simulink model "F16_Model_"  (R2025b)
settings: Solver=VariableStepAuto  StartTime=0.0  StopTime=100  RelTol=1e-3
values from neighbouring files (symbols this model uses):
  aero_data =     [aero_data.mat]
  b = 9.144    [initialization.m]
  c_bar = 3.45    [initialization.m]
  g = 9.81    [initialization.m]
  initial_pow = 50    [controlInputs.m]
  mass = 9295.4128    [initialization.m]
  S = 27.87    [initialization.m]
  u1 = 0    [controlInputs.m]
  u2 = 0    [controlInputs.m]
  u3 = -2    [controlInputs.m]
  u4 = 0    [controlInputs.m]
  u5 = 0    [controlInputs.m]
  u6 = 0.6    [controlInputs.m]
  xcg = 0.3*c_bar    (= 1.035)    [initialization.m]
  xcgr = 0.35*c_bar    (= 1.2075)    [initialization.m]
libraries: simulink_extras x9, aerolibfltsims x2, aerolibobsolete x1
(part 1 of 2)
settings Model: Creator=deepa  LastModifiedBy=deepa

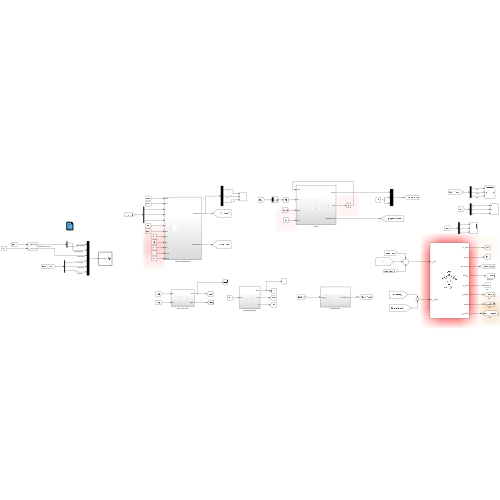
[thumbnail: Simulink's stored preview of the top-level diagram]
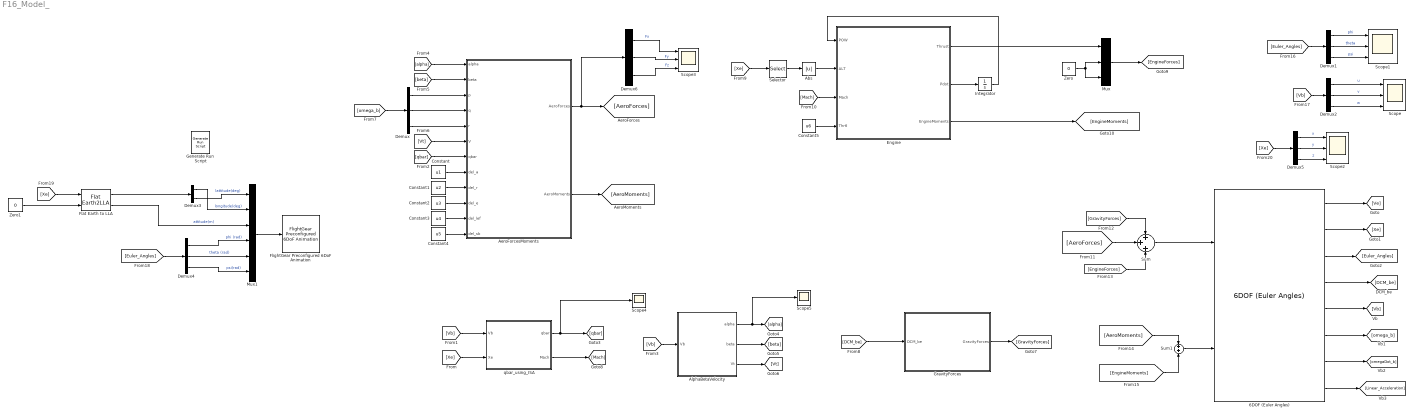
== system F16_Model_ ==
  6DOF (Euler Angles) : aerolibobsolete/6DOF (Euler Angles)  units=Metric (MKS)  mtype=Fixed  rep=Euler Angles  xme_0=[0 0 -1000]  Vm_0=[100 0 0]  eul_0=[0 0 0]  pm_0=[0 0 0]  mass_0=mass  mass_e=0.5  mass_f=2.0  inertia=I  inertia_e=eye(3)  inertia_f=2*eye(3)  k_quat=1.0  vre_flag=on  abi_flag=off  aMode=0  xme_statename=''  Vm_statename=''  eul_statename=''  quat_statename=''  pm_statename=''  mass_statename=''
  Abs : Abs  SaturateOnIntegerOverflow=off
  AeroForcesMoments : Subsystem
  AlphaBetaVelocity : Subsystem
  Constant : Constant  Value=u1
  Constant1 : Constant  Value=u2
  Constant2 : Constant  Value=u3
  Constant3 : Constant  Value=u4
  Constant4 : Constant  Value=u5
  Constant5 : Constant  Value=u6
  Demux{,1..2,4..6} (6 alike) : Demux  Outputs=3
  Demux3 : Demux  Outputs=2
  Engine : Subsystem
  Flat Earth to LLA : FlatEarth2LLA  R=6378137
  FlightGear Preconfigured 6DoF Animation : aerolibfltsims/FlightGear Preconfigured 6DoF Animation  xFlightGearVersion=v2019.1  DestinationIpAddress=127.0.0.1  DestinationPort=5502  SampleTime=1/30  packetVersion=24
  Generate Run Script : aerolibfltsims/Generate Run Script  Architecture=Win64  dataFlow=Send  GeometryModelName=c172p  AirportId=KSFO  RunwayId=10L  InitialAltitude=7224  InitialHeading=113  OffsetDistance=4.72  OffsetAzimuth=0  InstallScenery=off  DisableShaders=on  OriginAddress=127.0.0.1  DestinationPort=5502  OriginPort=5505  LocalAddress=127.0.0.1  OutputFileName=runfg.bat  FlightGearBaseDirectory=C:\Program Files\FlightGear 2024.1
  GravityForces : Subsystem
  Integrator : Integrator  InitialCondition=initial_pow
  Mux : Mux  Inputs=3
  Mux1 : Mux  Inputs=6
  Scope{,1..3} (4 alike) : Scope  NumInputPorts=3
      Scope settings: ActiveDisplayYMinimum=-502.98188581744421  ActiveDisplayYMaximum=2375.231294084077
      Scope1 settings: ActiveDisplayYMinimum=-1.0905728605767717  ActiveDisplayYMaximum=2.3543796241873545
      Scope2 settings: ActiveDisplayYMinimum=-88303.697025935631  ActiveDisplayYMaximum=46323.817378963853
      Scope3 settings: ActiveDisplayYMinimum=-6.05748400595E+6  ActiveDisplayYMaximum=3.40196349632E+6
  Scope4 : Scope
      settings: ActiveDisplayYMinimum=-166166.62177  ActiveDisplayYMaximum=1.49575944273E+6  DataLoggingVariableName=ScopeData2
  Scope5 : Scope
      settings: ActiveDisplayYMinimum=-7.38258  ActiveDisplayYMaximum=1.95471  DataLoggingVariableName=ScopeData3
  Selector : Selector  InputPortWidth=3  IndexOptions=Index vector (dialog)  Indices=3  OutputSizes=1
  Sum : Sum  Inputs=+++
  Sum1 : Sum
  Zero : Constant  Value=0  OutDataTypeStr=Inherit: Inherit via back propagation
  Zero1 : Constant  Value=0  OutDataTypeStr=Inherit: Inherit via back propagation
  qbar_using_ISA : Subsystem
  wires:
  6DOF (Euler Angles)/8 -> [Linear_Acceleration]
  6DOF (Euler Angles)/1 -> [Ve]
  6DOF (Euler Angles)/2 -> [Xe]
  6DOF (Euler Angles)/3 -> [Euler_Angles]
  6DOF (Euler Angles)/4 -> [DCM_be]
  6DOF (Euler Angles)/5 -> [Vb]
  6DOF (Euler Angles)/6 -> [omega_b]
  6DOF (Euler Angles)/7 -> [omegaDot_b]
  [Xe] -> qbar_using_ISA/2(Xe)
  [Vb] -> qbar_using_ISA/1(Vb)
  qbar_using_ISA/1(qbar) -> Scope4/1, [qbar]
  [qbar] -> AeroForcesMoments/7(qbar)
  [Vb] -> AlphaBetaVelocity/1(Vb)
  AlphaBetaVelocity/1(alpha) -> Scope5/1, [alpha]
  AlphaBetaVelocity/2(beta) -> [beta]
  AlphaBetaVelocity/3(Vt) -> [Vt]
  [alpha] -> AeroForcesMoments/1(alpha)
  [beta] -> AeroForcesMoments/2(beta)
  [Vt] -> AeroForcesMoments/6(V)
  [omega_b] -> Demux/1
  Demux/1 -> AeroForcesMoments/3(p)
  Demux/2 -> AeroForcesMoments/4(q)
  Demux/3 -> AeroForcesMoments/5(r)
  [DCM_be] -> GravityForces/1(DCM_be)
  GravityForces/1(GravityForces) -> [GravityForces]
  Engine/2(Pdot) -> Integrator/1
  Integrator/1 -> Engine/1(POW)
  [Xe] -> Selector/1
  Selector/1 -> Abs/1
  Abs/1 -> Engine/2(ALT)
  qbar_using_ISA/2(Mach) -> [Mach]
  [Mach] -> Engine/3(Mach)
  Engine/1(Thrust) -> Mux/1
  Mux/1 -> [EngineForces]
  Zero/1 -> Mux/2, Mux/3
  AeroForcesMoments/1(AeroForces) -> Demux6/1, [AeroForces]
  AeroForcesMoments/2(AeroMoments) -> [AeroMoments]
  [EngineForces] -> Sum/3
  [AeroForces] -> Sum/2
  [GravityForces] -> Sum/1
  Sum/1 -> 6DOF (Euler Angles)/1
  Engine/3(EngineMoments) -> [EngineMoments]
  [EngineMoments] -> Sum1/2
  [AeroMoments] -> Sum1/1
  Sum1/1 -> 6DOF (Euler Angles)/2
  Constant/1 -> AeroForcesMoments/8(del_a)
  Constant1/1 -> AeroForcesMoments/9(del_r)
  Constant2/1 -> AeroForcesMoments/10(del_e)
  Constant3/1 -> AeroForcesMoments/11(del_lef)
  Constant4/1 -> AeroForcesMoments/12(del_sb)
  Constant5/1 -> Engine/4(Thrtl)
  [Euler_Angles] -> Demux1/1
  Demux1/1 -> Scope1/1  "phi"
  Demux1/2 -> Scope1/2  "theta"
  Demux1/3 -> Scope1/3  "psi"
  [Vb] -> Demux2/1
  Demux2/1 -> Scope/1  "u"
  Demux2/2 -> Scope/2  "v"
  Demux2/3 -> Scope/3  "w"
  Flat Earth to LLA/1 -> Demux3/1
  Demux3/2 -> Mux1/1  "lattitude(deg)"
  Demux3/1 -> Mux1/2  "longitude(deg)"
  Flat Earth to LLA/2 -> Mux1/3  "attitude(m)"
  Demux4/1 -> Mux1/4  "phi (rad)"
  Demux4/2 -> Mux1/5  "theta (rad)"
  Demux4/3 -> Mux1/6  "psi(rad)"
  [Euler_Angles] -> Demux4/1
  Mux1/1 -> FlightGear Preconfigured 6DoF Animation/1
  [Xe] -> Flat Earth to LLA/1
  Zero1/1 -> Flat Earth to LLA/2
  [Xe] -> Demux5/1
  Demux5/1 -> Scope2/1  "x"
  Demux5/2 -> Scope2/2  "y"
  Demux5/3 -> Scope2/3  "z"
  Demux6/1 -> Scope3/1  "Fx"
  Demux6/2 -> Scope3/2  "Fy"
  Demux6/3 -> Scope3/3  "Fz"

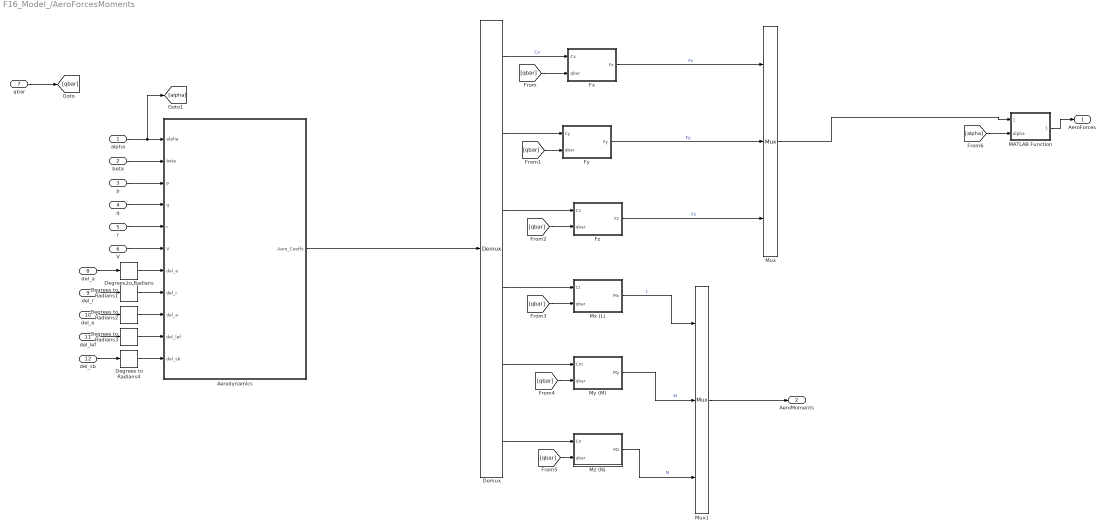
== system F16_Model_/AeroForcesMoments ==
  alpha : Inport
  beta : Inport  Port=2
  p : Inport  Port=3
  q : Inport  Port=4
  r : Inport  Port=5
  V : Inport  Port=6
  qbar : Inport  Port=7
  del_a : Inport  Port=8
  del_r : Inport  Port=9
  del_e : Inport  Port=10
  del_lef : Inport  Port=11
  del_sb : Inport  Port=12
  Aerodynamics : Subsystem
      mask Display: image('plane-8107709.jpg', [20,20,20,20,100,100]);
  Degrees to Radians{,1..4} (5 alike) : simulink_extras/Transformations/Degrees to Radians
  Demux : Demux  Outputs=6
  Fx : Subsystem
  Fy : Subsystem
  Fz : Subsystem
  MATLAB Function : MATLAB Function  TreatAsAtomicUnit=on
  Mux : Mux  Inputs=3
  Mux1 : Mux  Inputs=3
  Mx (L) : Subsystem
  My (M) : Subsystem
  Mz (N) : Subsystem
  AeroForces : Outport
  AeroMoments : Outport  Port=2
  wires:
  Aerodynamics/1(Aero_Coeffs) -> Demux/1
  Demux/3 -> Fz/1(Cz)
  Demux/5 -> My (M)/1(Cm)
  Demux/6 -> Mz (N)/1(Cn)
  Demux/2 -> Fy/1(Cy)
  Demux/4 -> Mx (L)/1(Cl)
  qbar/1 -> [qbar]
  Demux/1 -> Fx/1(Cx)  "Cx"
  Fx/1(Fx) -> Mux/1  "Fx"
  [qbar] -> Fx/2(qbar)
  [qbar] -> Fy/2(qbar)
  [qbar] -> Fz/2(qbar)
  [qbar] -> Mx (L)/2(qbar)
  [qbar] -> My (M)/2(qbar)
  [qbar] -> Mz (N)/2(qbar)
  Mx (L)/1(Mx) -> Mux1/1  "L"
  My (M)/1(My) -> Mux1/2  "M"
  Mz (N)/1(Mz) -> Mux1/3  "N"
  Mux/1 -> MATLAB Function/1(F_stability)
  Mux1/1 -> AeroMoments/1
  alpha/1 -> [alpha], Aerodynamics/1(alpha)
  beta/1 -> Aerodynamics/2(beta)
  p/1 -> Aerodynamics/3(p)
  q/1 -> Aerodynamics/4(q)
  r/1 -> Aerodynamics/5(r)
  V/1 -> Aerodynamics/6(V)
  del_a/1 -> Degrees to Radians/1
  del_r/1 -> Degrees to Radians1/1
  del_e/1 -> Degrees to Radians2/1
  del_lef/1 -> Degrees to Radians3/1
  del_sb/1 -> Degrees to Radians4/1
  Degrees to Radians/1 -> Aerodynamics/7(del_a)
  Degrees to Radians1/1 -> Aerodynamics/8(del_r)
  Degrees to Radians2/1 -> Aerodynamics/9(del_e)
  Degrees to Radians3/1 -> Aerodynamics/10(del_lef)
  Degrees to Radians4/1 -> Aerodynamics/11(del_sb)
  Fy/1(Fy) -> Mux/2  "Fy"
  Fz/1(Fz) -> Mux/3  "Fz"
  MATLAB Function/1(F_body) -> AeroForces/1
  [alpha] -> MATLAB Function/2(alpha)

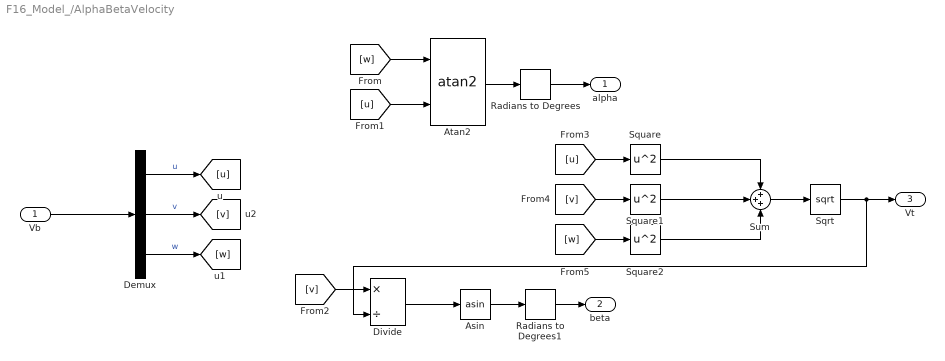
== system F16_Model_/AlphaBetaVelocity ==
  Vb : Inport
  Asin : Trigonometry  Operator=asin
  Atan2 : Trigonometry  Operator=atan2
  Demux : Demux  Outputs=3
  Divide : Product  Inputs=*/
  Radians to Degrees : simulink_extras/Transformations/Radians to Degrees
  Radians to Degrees1 : simulink_extras/Transformations/Radians to Degrees
  Sqrt : Sqrt
  Square : Math  Operator=square
  Square1 : Math  Operator=square
  Square2 : Math  Operator=square
  Sum : Sum  Inputs=+++
  alpha : Outport
  beta : Outport  Port=2
  Vt : Outport  Port=3
  wires:
  Vb/1 -> Demux/1
  Demux/1 -> [u]  "u"
  Demux/2 -> [v]  "v"
  Demux/3 -> [w]  "w"
  [u] -> Atan2/2
  [w] -> Atan2/1
  Atan2/1 -> Radians to Degrees/1
  [v] -> Divide/1
  Divide/1 -> Asin/1
  [u] -> Square/1
  [v] -> Square1/1
  [w] -> Square2/1
  Square/1 -> Sum/1
  Square1/1 -> Sum/2
  Square2/1 -> Sum/3
  Sum/1 -> Sqrt/1
  Sqrt/1 -> Divide/2, Vt/1
  Radians to Degrees/1 -> alpha/1
  Radians to Degrees1/1 -> beta/1
  Asin/1 -> Radians to Degrees1/1

== system F16_Model_/Engine ==
  POW : Inport
  ALT : Inport  Port=2
  Mach : Inport  Port=3
  Thrtl : Inport  Port=4
  Mux : Mux  Inputs=3
  PDOT : MATLAB Function  TreatAsAtomicUnit=on
  TGEAR : MATLAB Function  TreatAsAtomicUnit=on
  Thrust_ : MATLAB Function  TreatAsAtomicUnit=on
  Zero : Constant  Value=0  OutDataTypeStr=Inherit: Inherit via back propagation
  Thrust : Outport
  Pdot : Outport  Port=2
  EngineMoments : Outport  Port=3
  wires:
  Mach/1 -> Thrust_/3(MACH)
  POW/1 -> PDOT/1(P3), Thrust_/1(POW)
  Thrtl/1 -> TGEAR/1(THTL)
  TGEAR/1(TGEAR) -> PDOT/2(P1)
  PDOT/1(PDOT) -> Pdot/1
  ALT/1 -> Thrust_/2(ALT)
  Zero/1 -> Mux/3, Mux/2, Mux/1
  Mux/1 -> EngineMoments/1
  Thrust_/1(THRUST) -> Thrust/1

== system F16_Model_/GravityForces ==
  DCM_be : Inport
  Constant : Constant  Value=g
  Constant1 : Constant  Value=0
  Gain : Gain  Gain=mass
  Mux : Mux  Inputs=3
  Product : Product  Multiplication=Matrix(*)
  GravityForces : Outport
  wires:
  Constant/1 -> Gain/1
  Gain/1 -> Mux/3
  Constant1/1 -> Mux/2, Mux/1
  Mux/1 -> Product/2  "3x1"
  DCM_be/1 -> Product/1  "3x3"
  Product/1 -> GravityForces/1

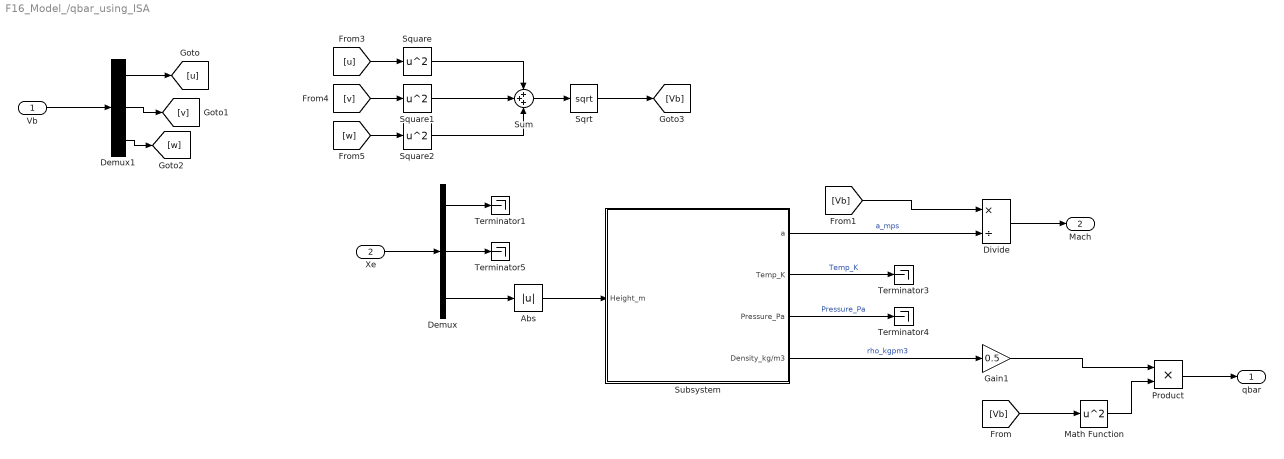
== system F16_Model_/qbar_using_ISA ==
  Vb : Inport
  Xe : Inport  Port=2
  Abs : Abs  SaturateOnIntegerOverflow=off
  Demux : Demux  Outputs=3
  Demux1 : Demux  Outputs=3
  Divide : Product  Inputs=*/
  Gain1 : Gain  Gain=0.5
  Math Function : Math  Operator=square
  Product : Product
  Sqrt : Sqrt
  Square : Math  Operator=square
  Square1 : Math  Operator=square
  Square2 : Math  Operator=square
  Subsystem : Subsystem
  Sum : Sum  Inputs=+++
  Terminator{1,3..5} (4 alike) : Terminator
  qbar : Outport
  Mach : Outport  Port=2
  wires:
  Subsystem/4(Density_kg/m3) -> Gain1/1  "rho_kgpm3"
  Subsystem/1(a) -> Divide/2  "a_mps"
  Subsystem/2(Temp_K) -> Terminator3/1  "Temp_K"
  Subsystem/3(Pressure_Pa) -> Terminator4/1  "Pressure_Pa"
  Gain1/1 -> Product/1
  Math Function/1 -> Product/2
  Product/1 -> qbar/1
  Xe/1 -> Demux/1
  Demux/1 -> Terminator1/1
  Demux/2 -> Terminator5/1
  Demux/3 -> Abs/1
  Vb/1 -> Demux1/1
  [Vb] -> Math Function/1
  [Vb] -> Divide/1
  Divide/1 -> Mach/1
  [v] -> Square1/1
  [w] -> Square2/1
  [u] -> Square/1
  Sum/1 -> Sqrt/1
  Square2/1 -> Sum/3
  Square/1 -> Sum/1
  Square1/1 -> Sum/2
  Sqrt/1 -> [Vb]
  Demux1/1 -> [u]
  Demux1/2 -> [v]
  Demux1/3 -> [w]
  Abs/1 -> Subsystem/1(Height_m)

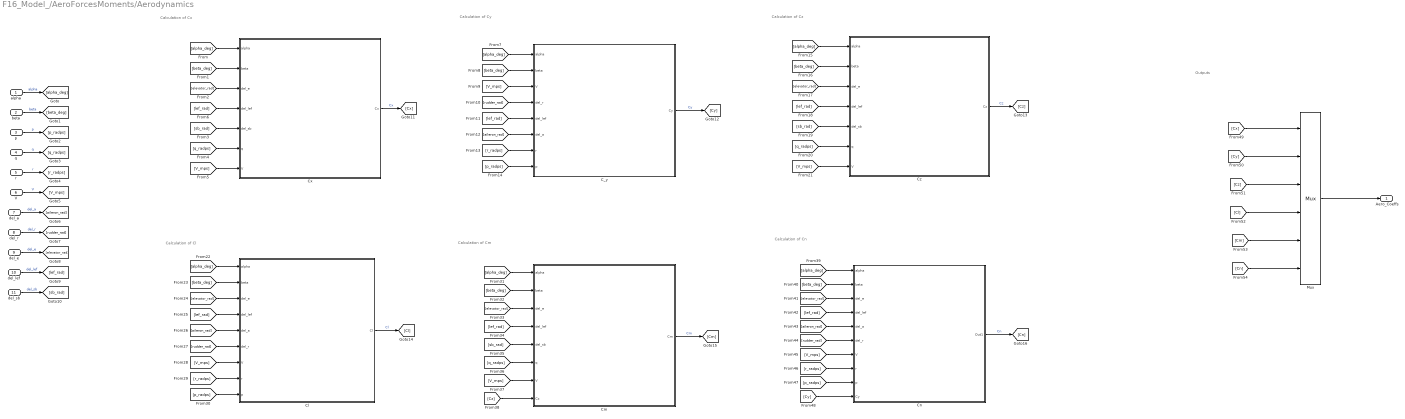
== system F16_Model_/AeroForcesMoments/Aerodynamics ==
  note: Outputs
  note: Calculation of Cn
  note: Calculation of Cm
  note: Calculation of Cl
  note: Calculation of Cy
  note: Calculation of Cx
  note: Calculation of Cz
  alpha : Inport
  beta : Inport  Port=2
  p : Inport  Port=3
  q : Inport  Port=4
  r : Inport  Port=5
  V : Inport  Port=6
  del_a : Inport  Port=7
  del_r : Inport  Port=8
  del_e : Inport  Port=9
  del_lef : Inport  Port=10
  del_sb : Inport  Port=11
  C_y : Subsystem
  Cl : Subsystem
  Cm : Subsystem
  Cn : Subsystem
  Cx : Subsystem
  Cz : Subsystem
  Mux : Mux  Inputs=6
  Aero_Coeffs : Outport
  wires:
  Mux/1 -> Aero_Coeffs/1
  alpha/1 -> [alpha_deg]  "alpha"
  beta/1 -> [beta_deg]  "beta"
  p/1 -> [p_radps]  "p"
  q/1 -> [q_radps]  "q"
  r/1 -> [r_radps]  "r"
  V/1 -> [V_mps]  "V"
  del_a/1 -> [aileron_rad]  "del_a"
  del_r/1 -> [rudder_rad]  "del_r"
  del_e/1 -> [elevator_rad]  "del_e"
  del_lef/1 -> [lef_rad]  "del_lef"
  del_sb/1 -> [sb_rad]  "del_sb"
  [alpha_deg] -> Cx/1(alpha)
  [beta_deg] -> Cx/2(beta)
  [elevator_rad] -> Cx/3(del_e)
  [lef_rad] -> Cx/4(del_lef)
  [sb_rad] -> Cx/5(del_sb)
  [q_radps] -> Cx/6(q)
  [V_mps] -> Cx/7(V)
  Cx/1(Cx) -> [Cx]  "Cx"
  [alpha_deg] -> C_y/1(alpha)
  [beta_deg] -> C_y/2(beta)
  [V_mps] -> C_y/3(V)
  [rudder_rad] -> C_y/4(del_r)
  [lef_rad] -> C_y/5(del_lef)
  [aileron_rad] -> C_y/6(del_a)
  [r_radps] -> C_y/7(r)
  [p_radps] -> C_y/8(p)
  C_y/1(Cy) -> [Cy]  "Cy"
  [alpha_deg] -> Cz/1(alpha)
  [beta_deg] -> Cz/2(beta)
  [elevator_rad] -> Cz/3(del_e)
  [lef_rad] -> Cz/4(del_lef)
  [sb_rad] -> Cz/5(del_sb)
  [q_radps] -> Cz/6(q)
  [V_mps] -> Cz/7(V)
  Cz/1(Cz) -> [Cz]  "Cz"
  [alpha_deg] -> Cl/1(alpha)
  [beta_deg] -> Cl/2(beta)
  [elevator_rad] -> Cl/3(del_e)
  [lef_rad] -> Cl/4(del_lef)
  [aileron_rad] -> Cl/5(del_a)
  [rudder_rad] -> Cl/6(del_r)
  [V_mps] -> Cl/7(V)
  [r_radps] -> Cl/8(r)
  [p_radps] -> Cl/9(p)
  Cl/1(Cl) -> [Cl]  "Cl"
  [alpha_deg] -> Cm/1(alpha)
  [beta_deg] -> Cm/2(beta)
  [elevator_rad] -> Cm/3(del_e)
  [lef_rad] -> Cm/4(del_lef)
  [sb_rad] -> Cm/5(del_sb)
  [q_radps] -> Cm/6(q)
  [V_mps] -> Cm/7(V)
  [Cz] -> Cm/8(Cz)
  Cm/1(Cm) -> [Cm]  "Cm"
  [alpha_deg] -> Cn/1(alpha)
  [beta_deg] -> Cn/2(beta)
  [elevator_rad] -> Cn/3(del_e)
  [lef_rad] -> Cn/4(del_lef)
  [aileron_rad] -> Cn/5(del_a)
  [rudder_rad] -> Cn/6(del_r)
  [V_mps] -> Cn/7(V)
  [r_radps] -> Cn/8(r)
  [p_radps] -> Cn/9(p)
  [Cy] -> Cn/10(Cy)
  Cn/1(Out1) -> [Cn]  "Cn"
  [Cx] -> Mux/1
  [Cy] -> Mux/2
  [Cz] -> Mux/3
  [Cl] -> Mux/4
  [Cm] -> Mux/5
  [Cn] -> Mux/6

== system F16_Model_/AeroForcesMoments/Fx ==
  Cx : Inport
  qbar : Inport  Port=2
  Gain : Gain  Gain=S
  Product : Product
  Fx : Outport
  wires:
  Product/1 -> Fx/1
  Gain/1 -> Product/1
  qbar/1 -> Product/2
  Cx/1 -> Gain/1

== system F16_Model_/AeroForcesMoments/Fy ==
  Cy : Inport
  qbar : Inport  Port=2
  Gain : Gain  Gain=S
  Product : Product
  Fy : Outport
  wires:
  Cy/1 -> Gain/1
  qbar/1 -> Product/2
  Gain/1 -> Product/1
  Product/1 -> Fy/1

== system F16_Model_/AeroForcesMoments/Fz ==
  Cz : Inport
  qbar : Inport  Port=2
  Gain : Gain  Gain=S
  Product : Product
  Fz : Outport
  wires:
  Product/1 -> Fz/1
  Gain/1 -> Product/1
  qbar/1 -> Product/2
  Cz/1 -> Gain/1

== system F16_Model_/AeroForcesMoments/Mx (L) ==
  Cl : Inport
  qbar : Inport  Port=2
  Gain : Gain  Gain=S*b
  Product : Product
  Mx : Outport
  wires:
  Cl/1 -> Gain/1
  qbar/1 -> Product/2
  Gain/1 -> Product/1
  Product/1 -> Mx/1

== system F16_Model_/AeroForcesMoments/My (M) ==
  Cm : Inport
  qbar : Inport  Port=2
  Gain : Gain  Gain=S*c_bar
  Product : Product
  My : Outport
  wires:
  Product/1 -> My/1
  Gain/1 -> Product/1
  qbar/1 -> Product/2
  Cm/1 -> Gain/1

== system F16_Model_/AeroForcesMoments/Mz (N) ==
  Cn : Inport
  qbar : Inport  Port=2
  Gain : Gain  Gain=S*b
  Product : Product
  Mz : Outport
  wires:
  Cn/1 -> Gain/1
  qbar/1 -> Product/2
  Gain/1 -> Product/1
  Product/1 -> Mz/1

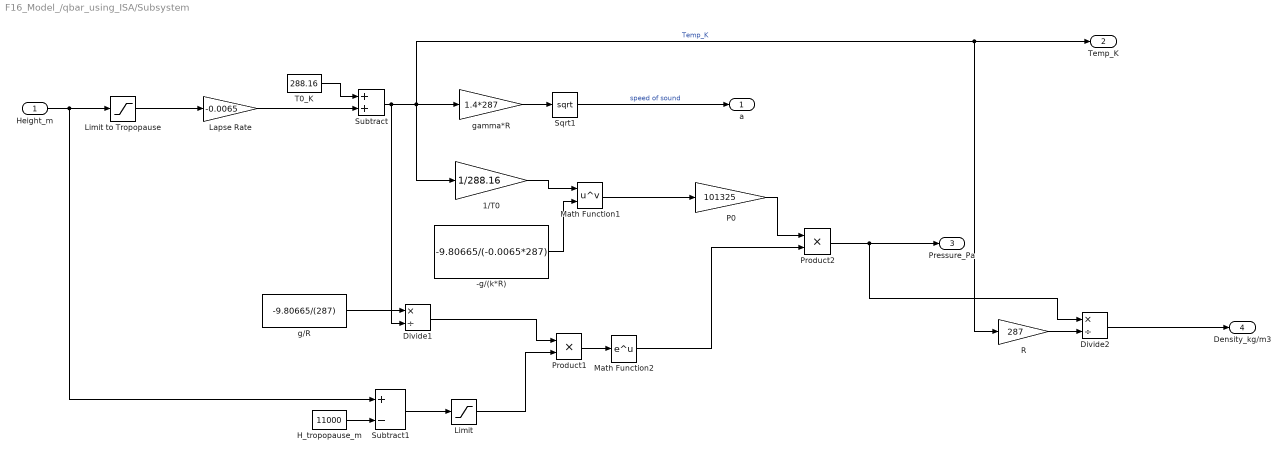
== system F16_Model_/qbar_using_ISA/Subsystem ==
  Height_m : Inport
  -g/(k*R) : Constant  Value=-9.80665/(-0.0065*287)
  1/T0 : Gain  Gain=1/288.16
  Divide1 : Product  Inputs=*/
  Divide2 : Product  Inputs=*/
  H_tropopause_m : Constant  Value=11000
  Lapse Rate : Gain  Gain=-0.0065
  "Limit " : Saturate  UpperLimit=inf  LowerLimit=0
  Limit to Tropopause : Saturate  UpperLimit=11000  LowerLimit=0
  Math Function1 : Math  Operator=pow
  Math Function2 : Math
  P0 : Gain  Gain=101325
  Product1 : Product
  Product2 : Product
  "R " : Gain  Gain=287
  Sqrt1 : Sqrt
  Subtract : Sum
  Subtract1 : Sum  Inputs=+-
  T0_K : Constant  Value=288.16
  g/R : Constant  Value=-9.80665/(287)
  gamma*R : Gain  Gain=1.4*287
  a : Outport
  Temp_K : Outport  Port=2
  Pressure_Pa : Outport  Port=3
  Density_kg/m3 : Outport  Port=4
  wires:
  1/T0/1 -> Math Function1/1
  H_tropopause_m/1 -> Subtract1/2
  P0/1 -> Product2/1
  Subtract/1 -> Divide1/2, gamma*R/1, 1/T0/1, Temp_K/1, "R "/1  "Temp_K"
  Lapse Rate/1 -> Subtract/2
  "R "/1 -> Divide2/2
  gamma*R/1 -> Sqrt1/1
  Limit to Tropopause/1 -> Lapse Rate/1
  T0_K/1 -> Subtract/1
  g/R/1 -> Divide1/1
  Product1/1 -> Math Function2/1
  Divide1/1 -> Product1/1
  Sqrt1/1 -> a/1  "speed of sound"
  Math Function1/1 -> P0/1
  Divide2/1 -> Density_kg/m3/1
  Product2/1 -> Pressure_Pa/1, Divide2/1
  Subtract1/1 -> "Limit "/1
  Height_m/1 -> Subtract1/1, Limit to Tropopause/1
  -g/(k*R)/1 -> Math Function1/2
  "Limit "/1 -> Product1/2
  Math Function2/1 -> Product2/2

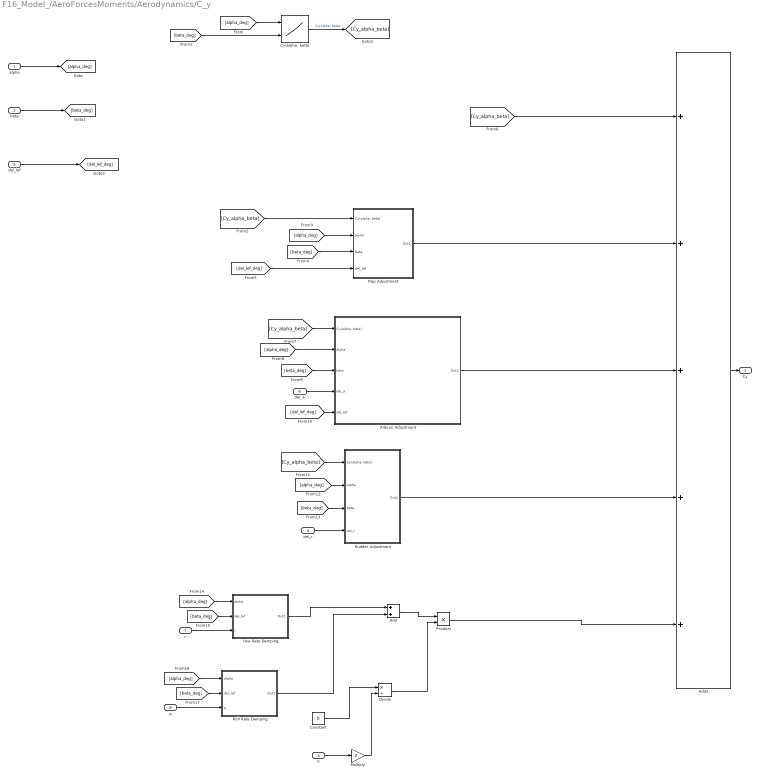
== system F16_Model_/AeroForcesMoments/Aerodynamics/C_y ==
  alpha : Inport
  beta : Inport  Port=2
  V : Inport  Port=3
  del_r : Inport  Port=4
  del_lef : Inport  Port=5
  del_a : Inport  Port=6
  r : Inport  Port=7
  p : Inport  Port=8
  Add : Sum
  Add2 : Sum  Inputs=+++++
  Aileron Adjustment : Subsystem
  Constant : Constant  Value=b
  "Cy(alpha, beta)" : Lookup_n-D  BreakpointsForDimension1=[-20, -15, -10, -5, 0, 5, 10, 15, 20, 25, 30, 35, 40, 45, 50, 55, 60, 70, 80, 90];  BreakpointsForDimension2=[-30, -25, -20, -15, -10, -8, -6, -4, -2, 0, 2, 4, 6, 8, 10, 15, 20, 25, 30];  Table=aero_data.Cy_alpha_beta  InternalRulePriority=Speed  RndMeth=Simplest
      settings: InputPortMap=u0,u1
  Divide : Product  Inputs=*/
  Flap Adjustment : Subsystem
  Multiply : Gain  Gain=2
  Product : Product
  Roll Rate Damping : Subsystem
  Rudder Adjustment : Subsystem
  Yaw Rate Damping : Subsystem
  Cy : Outport
  wires:
  Product/1 -> Add2/5
  Roll Rate Damping/1(Out1) -> Add/2
  Add/1 -> Product/1
  del_r/1 -> Rudder Adjustment/4(del_r)
  Yaw Rate Damping/1(Out1) -> Add/1
  p/1 -> Roll Rate Damping/3(p)
  Add2/1 -> Cy/1
  r/1 -> Yaw Rate Damping/3(r)
  del_a/1 -> Aileron Adjustment/4(del_a)
  Divide/1 -> Product/2
  Aileron Adjustment/1(Out1) -> Add2/3
  V/1 -> Multiply/1
  Flap Adjustment/1(Out1) -> Add2/2
  Rudder Adjustment/1(Out1) -> Add2/4
  Constant/1 -> Divide/1
  Multiply/1 -> Divide/2
  alpha/1 -> [alpha_deg]
  beta/1 -> [beta_deg]
  [alpha_deg] -> "Cy(alpha, beta)"/1
  [beta_deg] -> "Cy(alpha, beta)"/2
  "Cy(alpha, beta)"/1 -> [Cy_alpha_beta]  "Cy(alpha, beta)"
  [Cy_alpha_beta] -> Flap Adjustment/1("Cy(alpha, beta)")
  [alpha_deg] -> Flap Adjustment/2(alpha)
  [beta_deg] -> Flap Adjustment/3(beta)
  del_lef/1 -> [del_lef_deg]
  [del_lef_deg] -> Flap Adjustment/4(del_lef)
  [Cy_alpha_beta] -> Add2/1
  [Cy_alpha_beta] -> Aileron Adjustment/1("Cy(alpha, beta)")
  [alpha_deg] -> Aileron Adjustment/2(alpha)
  [beta_deg] -> Aileron Adjustment/3(beta)
  [del_lef_deg] -> Aileron Adjustment/5(del_lef)
  [Cy_alpha_beta] -> Rudder Adjustment/1("Cy(alpha, beta)")
  [alpha_deg] -> Rudder Adjustment/2(alpha)
  [beta_deg] -> Rudder Adjustment/3(beta)
  [alpha_deg] -> Yaw Rate Damping/1(alpha)
  [beta_deg] -> Yaw Rate Damping/2(del_lef)
  [alpha_deg] -> Roll Rate Damping/1(alpha)
  [beta_deg] -> Roll Rate Damping/2(del_lef)

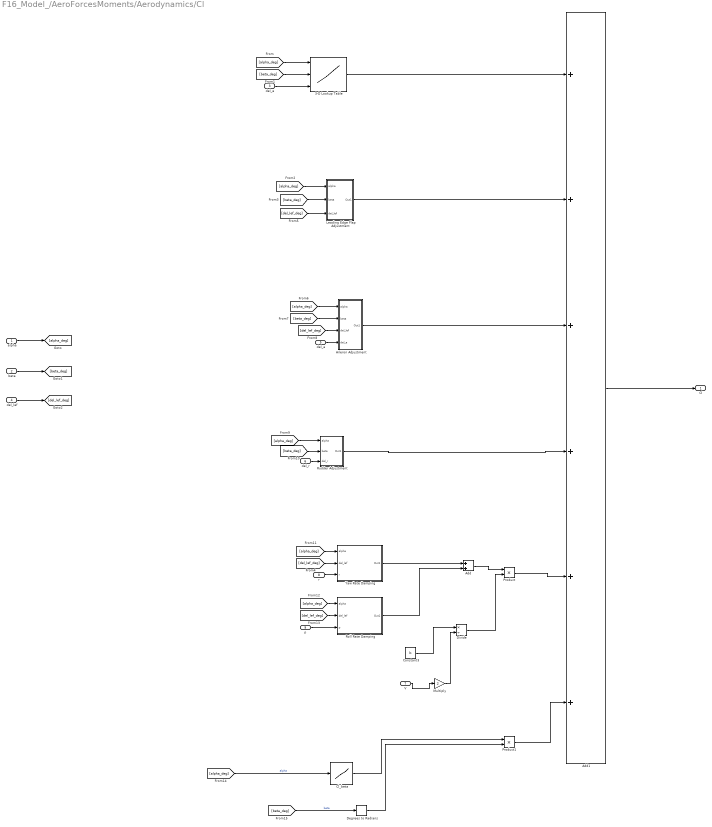
== system F16_Model_/AeroForcesMoments/Aerodynamics/Cl ==
  alpha : Inport
  beta : Inport  Port=2
  del_e : Inport  Port=3
  del_lef : Inport  Port=4
  del_a : Inport  Port=5
  del_r : Inport  Port=6
  V : Inport  Port=7
  r : Inport  Port=8
  p : Inport  Port=9
  3-D Lookup Table : Lookup_n-D  NumberOfTableDimensions=3  BreakpointsForDimension1=[-20, -15, -10, -5, 0, 5, 10, 15, 20, 25, 30, 35, 40, 45, 50, 55, 60, 70, 80, 90];  BreakpointsForDimension2=[-30, -25, -20, -15, -10, -8, -6, -4, -2, 0, 2, 4, 6, 8, 10, 15, 20, 25, 30];  BreakpointsForDimension3=[-25,0,25];  Table=aero_data.Cl_del_h  InternalRulePriority=Speed  RndMeth=Simplest
      settings: InputPortMap=u0,u1,u2
  Add : Sum
  Add1 : Sum  Inputs=++++++
  Aileron Adjustment : Subsystem
  Cl_beta : Lookup_n-D  NumberOfTableDimensions=1  BreakpointsForDimension1=[-20, -15, -10, -5, 0, 5, 10, 15, 20, 25, 30, 35, 40, 45, 50, 55, 60, 70, 80, 90];  Table=aero_data.del_Cl_beta  InternalRulePriority=Speed  RndMeth=Simplest
  Constant3 : Constant  Value=b
  Degrees to Radians : simulink_extras/Transformations/Degrees to Radians
  Divide : Product  Inputs=*/
  Leading Edge Flap Adjustment : Subsystem
  Multiply : Gain  Gain=2
  Product : Product
  Product1 : Product
  Roll Rate Damping : Subsystem
  Rudder Adjustment : Subsystem
  Yaw Rate Damping : Subsystem
  Cl : Outport
  wires:
  r/1 -> Yaw Rate Damping/3(r)
  Roll Rate Damping/1(Out1) -> Add/2
  del_r/1 -> Rudder Adjustment/3(del_r)
  Multiply/1 -> Divide/2
  Product/1 -> Add1/5
  p/1 -> Roll Rate Damping/3(p)
  del_a/1 -> Aileron Adjustment/4(del_a)
  3-D Lookup Table/1 -> Add1/1
  Constant3/1 -> Divide/1
  Rudder Adjustment/1(Out1) -> Add1/4
  Add1/1 -> Cl/1
  Leading Edge Flap Adjustment/1(Out1) -> Add1/2
  Yaw Rate Damping/1(Out1) -> Add/1
  Add/1 -> Product/1
  V/1 -> Multiply/1
  Divide/1 -> Product/2
  Cl_beta/1 -> Product1/1
  Degrees to Radians/1 -> Product1/2
  Product1/1 -> Add1/6
  [beta_deg] -> Degrees to Radians/1  "beta"
  [alpha_deg] -> Cl_beta/1  "alpha"
  alpha/1 -> [alpha_deg]
  beta/1 -> [beta_deg]
  [alpha_deg] -> 3-D Lookup Table/1
  [beta_deg] -> 3-D Lookup Table/2
  del_e/1 -> 3-D Lookup Table/3
  [alpha_deg] -> Leading Edge Flap Adjustment/1(alpha)
  [beta_deg] -> Leading Edge Flap Adjustment/2(beta)
  del_lef/1 -> [del_lef_deg]
  [del_lef_deg] -> Yaw Rate Damping/2(del_lef)
  [del_lef_deg] -> Leading Edge Flap Adjustment/3(del_lef)
  [alpha_deg] -> Aileron Adjustment/1(alpha)
  [beta_deg] -> Aileron Adjustment/2(beta)
  [del_lef_deg] -> Aileron Adjustment/3(del_lef)
  [alpha_deg] -> Rudder Adjustment/1(alpha)
  [beta_deg] -> Rudder Adjustment/2(beta)
  [alpha_deg] -> Yaw Rate Damping/1(alpha)
  [alpha_deg] -> Roll Rate Damping/1(alpha)
  [del_lef_deg] -> Roll Rate Damping/2(del_lef)
  Aileron Adjustment/1(Out1) -> Add1/3

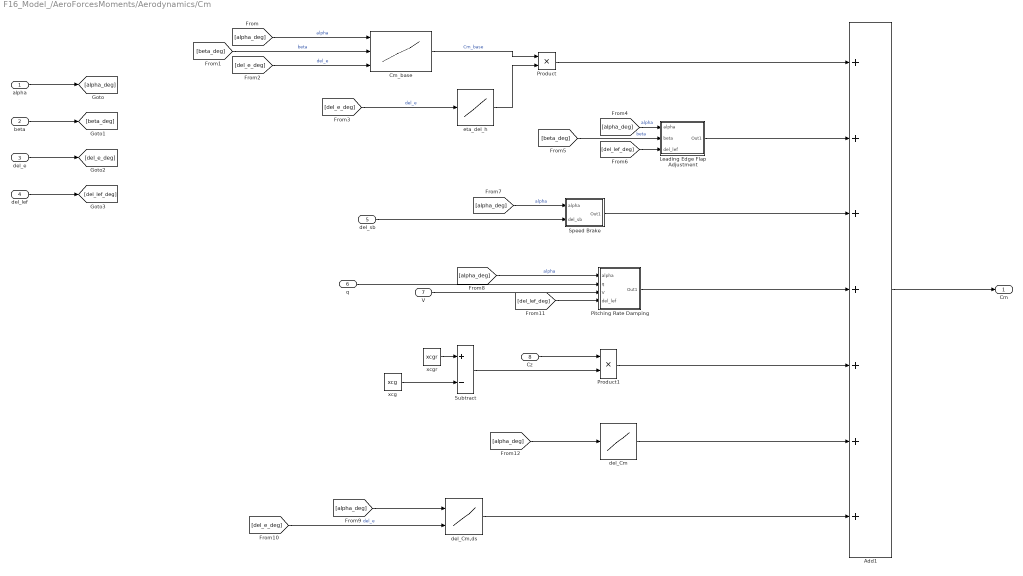
== system F16_Model_/AeroForcesMoments/Aerodynamics/Cm ==
  alpha : Inport
  beta : Inport  Port=2
  del_e : Inport  Port=3
  del_lef : Inport  Port=4
  del_sb : Inport  Port=5
  q : Inport  Port=6
  V : Inport  Port=7
  Cz : Inport  Port=8
  " Cm_base" : Lookup_n-D  NumberOfTableDimensions=3  BreakpointsForDimension1=[-20, -15, -10, -5, 0, 5, 10, 15, 20, 25, 30, 35, 40, 45, 50, 55, 60, 70, 80, 90];  BreakpointsForDimension2=[-30, -25, -20, -15, -10, -8, -6, -4, -2, 0, 2, 4, 6, 8, 10, 15, 20, 25, 30];  BreakpointsForDimension3=[-25, -10, 0, 10, 25]  Table=aero_data.Cm_del_h  InternalRulePriority=Speed  RndMeth=Simplest
      settings: InputPortMap=u0,u1,u2
  Add1 : Sum  Inputs=+++++++
  Leading Edge Flap Adjustment : Subsystem
  Pitching Rate Damping : Subsystem
  Product : Product
  Product1 : Product
  Speed Brake : Subsystem
  Subtract : Sum  Inputs=+-
  del_Cm : Lookup_n-D  NumberOfTableDimensions=1  BreakpointsForDimension1=[-20, -15, -10, -5, 0, 5, 10, 15, 20, 25, 30, 35, 40, 45, 50, 55, 60, 70, 80, 90]  Table=aero_data.del_Cm  InternalRulePriority=Speed  RndMeth=Simplest
  del_Cm,ds : Lookup_n-D  BreakpointsForDimension1=[-20, -15, -10, -5, 0, 5, 10, 15, 20, 25, 30, 35, 40, 45, 50, 55, 60, 70, 80, 90];  BreakpointsForDimension2=[-25, -10, 0, 10, 15, 20, 25]  Table=aero_data.del_Cm_ds  InternalRulePriority=Speed  RndMeth=Simplest
      settings: InputPortMap=u0,u1
  eta_del_h : Lookup_n-D  NumberOfTableDimensions=1  BreakpointsForDimension1=[-25, -10, 0, 10, 25]  Table=aero_data.eta_del_h  InternalRulePriority=Speed  RndMeth=Simplest
  xcg : Constant  Value=xcg
  xcgr : Constant  Value=xcgr
  Cm : Outport
  wires:
  Speed Brake/1(Out1) -> Add1/3
  Pitching Rate Damping/1(Out1) -> Add1/4
  Leading Edge Flap Adjustment/1(Out1) -> Add1/2
  Add1/1 -> Cm/1
  del_sb/1 -> Speed Brake/2(del_sb)
  q/1 -> Pitching Rate Damping/2(q)
  V/1 -> Pitching Rate Damping/3(V)
  " Cm_base"/1 -> Product/1  "Cm_base"
  eta_del_h/1 -> Product/2
  Product/1 -> Add1/1
  Cz/1 -> Product1/1
  xcgr/1 -> Subtract/1
  xcg/1 -> Subtract/2
  Subtract/1 -> Product1/2
  Product1/1 -> Add1/5
  del_Cm/1 -> Add1/6
  del_Cm,ds/1 -> Add1/7
  [alpha_deg] -> " Cm_base"/1  "alpha"
  [beta_deg] -> " Cm_base"/2  "beta"
  [del_e_deg] -> eta_del_h/1  "del_e"
  [del_e_deg] -> " Cm_base"/3  "del_e"
  alpha/1 -> [alpha_deg]
  beta/1 -> [beta_deg]
  del_e/1 -> [del_e_deg]
  del_lef/1 -> [del_lef_deg]
  [alpha_deg] -> Leading Edge Flap Adjustment/1(alpha)  "alpha"
  [beta_deg] -> Leading Edge Flap Adjustment/2(beta)  "beta"
  [del_lef_deg] -> Leading Edge Flap Adjustment/3(del_lef)
  [alpha_deg] -> Speed Brake/1(alpha)  "alpha"
  [alpha_deg] -> Pitching Rate Damping/1(alpha)  "alpha"
  [alpha_deg] -> del_Cm,ds/1
  [del_e_deg] -> del_Cm,ds/2  "del_e"
  [del_lef_deg] -> Pitching Rate Damping/4(del_lef)
  [alpha_deg] -> del_Cm/1

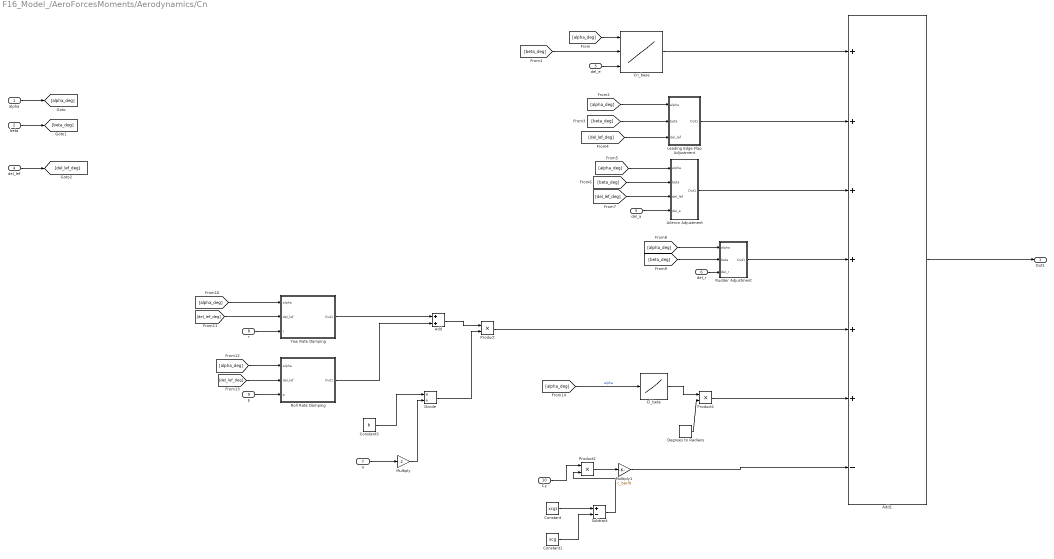
== system F16_Model_/AeroForcesMoments/Aerodynamics/Cn ==
  alpha : Inport
  beta : Inport  Port=2
  del_e : Inport  Port=3
  del_lef : Inport  Port=4
  del_a : Inport  Port=5
  del_r : Inport  Port=6
  V : Inport  Port=7
  r : Inport  Port=8
  p : Inport  Port=9
  Cy : Inport  Port=10
  Add : Sum
  Add1 : Sum  Inputs=++++++-
  Aileron Adjustment : Subsystem
  Cl_beta : Lookup_n-D  NumberOfTableDimensions=1  BreakpointsForDimension1=[-20, -15, -10, -5, 0, 5, 10, 15, 20, 25, 30, 35, 40, 45, 50, 55, 60, 70, 80, 90];  Table=aero_data.del_Cn_beta  InternalRulePriority=Speed  RndMeth=Simplest
  Cn_base : Lookup_n-D  NumberOfTableDimensions=3  BreakpointsForDimension1=[-20, -15, -10, -5, 0, 5, 10, 15, 20, 25, 30, 35, 40, 45, 50, 55, 60, 70, 80, 90];  BreakpointsForDimension2=[-30, -25, -20, -15, -10, -8, -6, -4, -2, 0, 2, 4, 6, 8, 10, 15, 20, 25, 30];  BreakpointsForDimension3=[-25,0,25];  Table=aero_data.Cn_del_h  InternalRulePriority=Speed  RndMeth=Simplest
      settings: InputPortMap=u0,u1,u2
  Constant : Constant  Value=xcgr
  Constant1 : Constant  Value=xcg
  Constant3 : Constant  Value=b
  Degrees to Radians : simulink_extras/Transformations/Degrees to Radians
  Divide : Product  Inputs=*/
  Leading Edge Flap Adjustment : Subsystem
  Multiply : Gain  Gain=2
  Multiply1 : Gain  Gain=c_bar/b
  Product : Product
  Product1 : Product
  Product2 : Product
  Roll Rate Damping : Subsystem
  Rudder Adjustment : Subsystem
  Subtract : Sum  Inputs=+-
  Yaw Rate Damping : Subsystem
  Out1 : Outport
  wires:
  r/1 -> Yaw Rate Damping/3(r)
  Roll Rate Damping/1(Out1) -> Add/2
  del_r/1 -> Rudder Adjustment/3(del_r)
  Aileron Adjustment/1(Out1) -> Add1/3
  Multiply/1 -> Divide/2
  Product/1 -> Add1/5
  p/1 -> Roll Rate Damping/3(p)
  del_a/1 -> Aileron Adjustment/4(del_a)
  Cn_base/1 -> Add1/1
  Constant3/1 -> Divide/1
  Rudder Adjustment/1(Out1) -> Add1/4
  Add1/1 -> Out1/1
  Leading Edge Flap Adjustment/1(Out1) -> Add1/2
  Yaw Rate Damping/1(Out1) -> Add/1
  del_e/1 -> Cn_base/3
  Add/1 -> Product/1
  V/1 -> Multiply/1
  Divide/1 -> Product/2
  Cl_beta/1 -> Product1/1
  Degrees to Radians/1 -> Product1/2
  Product1/1 -> Add1/6
  Constant/1 -> Subtract/1
  Constant1/1 -> Subtract/2
  Cy/1 -> Product2/1
  Subtract/1 -> Product2/2
  Product2/1 -> Multiply1/1
  Multiply1/1 -> Add1/7
  [alpha_deg] -> Cl_beta/1  "alpha"
  alpha/1 -> [alpha_deg]
  beta/1 -> [beta_deg]
  del_lef/1 -> [del_lef_deg]
  [alpha_deg] -> Cn_base/1
  [beta_deg] -> Cn_base/2
  [alpha_deg] -> Leading Edge Flap Adjustment/1(alpha)
  [beta_deg] -> Leading Edge Flap Adjustment/2(beta)
  [del_lef_deg] -> Leading Edge Flap Adjustment/3(del_lef)
  [alpha_deg] -> Aileron Adjustment/1(alpha)
  [beta_deg] -> Aileron Adjustment/2(beta)
  [del_lef_deg] -> Aileron Adjustment/3(del_lef)
  [alpha_deg] -> Rudder Adjustment/1(alpha)
  [beta_deg] -> Rudder Adjustment/2(beta)
  [alpha_deg] -> Yaw Rate Damping/1(alpha)
  [del_lef_deg] -> Yaw Rate Damping/2(del_lef)
  [alpha_deg] -> Roll Rate Damping/1(alpha)
  [del_lef_deg] -> Roll Rate Damping/2(del_lef)

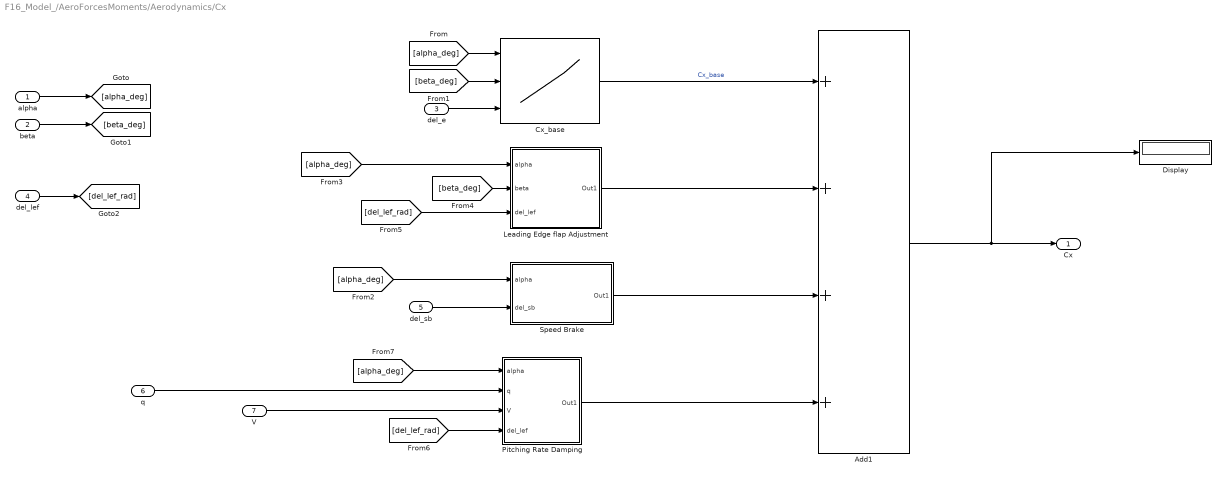
== system F16_Model_/AeroForcesMoments/Aerodynamics/Cx ==
  alpha : Inport
  beta : Inport  Port=2
  del_e : Inport  Port=3
  del_lef : Inport  Port=4
  del_sb : Inport  Port=5
  q : Inport  Port=6
  V : Inport  Port=7
  " Cx_base" : Lookup_n-D  NumberOfTableDimensions=3  BreakpointsForDimension1=[-20, -15, -10, -5, 0, 5, 10, 15, 20, 25, 30, 35, 40, 45, 50, 55, 60, 70, 80, 90];  BreakpointsForDimension2=[-30, -25, -20, -15, -10, -8, -6, -4, -2, 0, 2, 4, 6, 8, 10, 15, 20, 25, 30];  BreakpointsForDimension3=[-25, -10, 0, 10, 25];  Table=aero_data.Cx_del_h  InternalRulePriority=Speed  RndMeth=Simplest
      settings: InputPortMap=u0,u1,u2
  Add1 : Sum  Inputs=++++
  Display : Display
  Leading Edge flap Adjustment : Subsystem
  Pitching Rate Damping : Subsystem
  Speed Brake : Subsystem
  Cx : Outport
  wires:
  del_e/1 -> " Cx_base"/3
  Speed Brake/1(Out1) -> Add1/3
  " Cx_base"/1 -> Add1/1  "Cx_base"
  Pitching Rate Damping/1(Out1) -> Add1/4
  Leading Edge flap Adjustment/1(Out1) -> Add1/2
  Add1/1 -> Display/1, Cx/1
  del_sb/1 -> Speed Brake/2(del_sb)
  q/1 -> Pitching Rate Damping/2(q)
  V/1 -> Pitching Rate Damping/3(V)
  alpha/1 -> [alpha_deg]
  beta/1 -> [beta_deg]
  [alpha_deg] -> " Cx_base"/1
  [beta_deg] -> " Cx_base"/2
  del_lef/1 -> [del_lef_rad]
  [alpha_deg] -> Speed Brake/1(alpha)
  [alpha_deg] -> Leading Edge flap Adjustment/1(alpha)
  [beta_deg] -> Leading Edge flap Adjustment/2(beta)
  [del_lef_rad] -> Leading Edge flap Adjustment/3(del_lef)
  [del_lef_rad] -> Pitching Rate Damping/4(del_lef)
  [alpha_deg] -> Pitching Rate Damping/1(alpha)

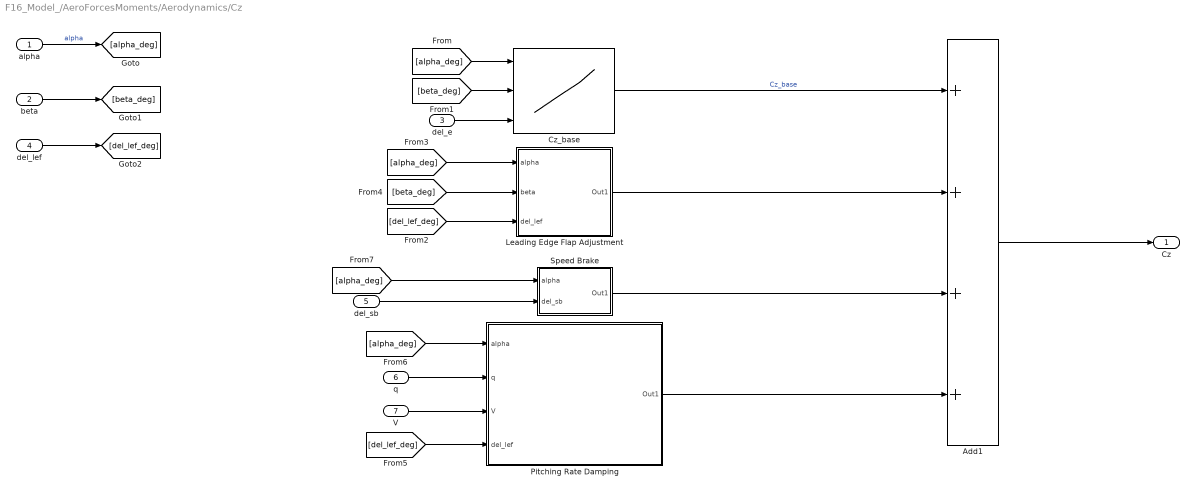
== system F16_Model_/AeroForcesMoments/Aerodynamics/Cz ==
  alpha : Inport
  beta : Inport  Port=2
  del_e : Inport  Port=3
  del_lef : Inport  Port=4
  del_sb : Inport  Port=5
  q : Inport  Port=6
  V : Inport  Port=7
  Add1 : Sum  Inputs=++++
  Cz_base : Lookup_n-D  NumberOfTableDimensions=3  BreakpointsForDimension1=[-20, -15, -10, -5, 0, 5, 10, 15, 20, 25, 30, 35, 40, 45, 50, 55, 60, 70, 80, 90];  BreakpointsForDimension2=[-30, -25, -20, -15, -10, -8, -6, -4, -2, 0, 2, 4, 6, 8, 10, 15, 20, 25, 30];  BreakpointsForDimension3=[-25, -10, 0, 10, 25];  Table=aero_data.Cz_del_h  InternalRulePriority=Speed  RndMeth=Simplest
      settings: InputPortMap=u0,u1,u2
  Leading Edge Flap Adjustment : Subsystem
  Pitching Rate Damping : Subsystem
  Speed Brake : Subsystem
  Cz : Outport
  wires:
  del_e/1 -> Cz_base/3
  Speed Brake/1(Out1) -> Add1/3
  Cz_base/1 -> Add1/1  "Cz_base"
  Pitching Rate Damping/1(Out1) -> Add1/4
  Leading Edge Flap Adjustment/1(Out1) -> Add1/2
  Add1/1 -> Cz/1
  del_sb/1 -> Speed Brake/2(del_sb)
  q/1 -> Pitching Rate Damping/2(q)
  V/1 -> Pitching Rate Damping/3(V)
  alpha/1 -> [alpha_deg]  "alpha"
  beta/1 -> [beta_deg]
  [alpha_deg] -> Cz_base/1
  [beta_deg] -> Cz_base/2
  del_lef/1 -> [del_lef_deg]
  [del_lef_deg] -> Leading Edge Flap Adjustment/3(del_lef)
  [alpha_deg] -> Leading Edge Flap Adjustment/1(alpha)
  [beta_deg] -> Leading Edge Flap Adjustment/2(beta)
  [del_lef_deg] -> Pitching Rate Damping/4(del_lef)
  [alpha_deg] -> Pitching Rate Damping/1(alpha)
  [alpha_deg] -> Speed Brake/1(alpha)

== system F16_Model_/AeroForcesMoments/Aerodynamics/C_y/Aileron Adjustment ==
  "Cy(alpha, beta)" : Inport
  alpha : Inport  Port=2
  beta : Inport  Port=3
  del_a : Inport  Port=4
  del_lef : Inport  Port=5
  Add1 : Sum
  Cy_del_a_20 : Lookup_n-D  BreakpointsForDimension1=[-20, -15, -10, -5, 0, 5, 10, 15, 20, 25, 30, 35, 40, 45, 50, 55, 60, 70, 80, 90];  BreakpointsForDimension2=[-30, -25, -20, -15, -10, -8, -6, -4, -2, 0, 2, 4, 6, 8, 10, 15, 20, 25, 30];  Table=aero_data.Cy_del_a_20  InternalRulePriority=Speed  RndMeth=Simplest
      settings: InputPortMap=u0,u1
  Multiply1 : Gain  Gain=0.05
  Product2 : Product
  Subtract1 : Sum  Inputs=-+
  del_Cy_del_a_20*(1-del_lef/25) : Subsystem
  Out1 : Outport
  wires:
  beta/1 -> Cy_del_a_20/2, del_Cy_del_a_20*(1-del_lef/25)/2(beta)
  Multiply1/1 -> Product2/2
  Add1/1 -> Product2/1
  Subtract1/1 -> Add1/1
  del_a/1 -> Multiply1/1
  Cy_del_a_20/1 -> Subtract1/2  "Cy_del_a_20"
  del_Cy_del_a_20*(1-del_lef/25)/1(Out1) -> Add1/2
  del_lef/1 -> del_Cy_del_a_20*(1-del_lef/25)/3(del_lef)
  Product2/1 -> Out1/1
  alpha/1 -> del_Cy_del_a_20*(1-del_lef/25)/1(alpha), Cy_del_a_20/1
  "Cy(alpha, beta)"/1 -> Subtract1/1

== system F16_Model_/AeroForcesMoments/Aerodynamics/C_y/Flap Adjustment ==
  "Cy(alpha, beta)" : Inport
  alpha : Inport  Port=2
  beta : Inport  Port=3
  del_lef : Inport  Port=4
  1-del_lef/25 : Subsystem
  Cy_lef : Lookup_n-D  BreakpointsForDimension1=[-20, -15, -10, -5, 0, 5, 10, 15, 20, 25, 30, 35, 40, 45];  BreakpointsForDimension2=[-30, -25, -20, -15, -10, -8, -6, -4, -2, 0, 2, 4, 6, 8, 10, 15, 20, 25, 30];  Table=aero_data.Cy_lef  InternalRulePriority=Speed  RndMeth=Simplest
      settings: InputPortMap=u0,u1
  Product3 : Product
  Subtract2 : Sum  Inputs=+-
  Out1 : Outport
  wires:
  "Cy(alpha, beta)"/1 -> Subtract2/2
  1-del_lef/25/1(1 - del_lef/25) -> Product3/2
  del_lef/1 -> 1-del_lef/25/1(del_lef1)
  Cy_lef/1 -> Subtract2/1  "Cy_lef"
  Subtract2/1 -> Product3/1
  alpha/1 -> Cy_lef/1
  beta/1 -> Cy_lef/2
  Product3/1 -> Out1/1

== system F16_Model_/AeroForcesMoments/Aerodynamics/C_y/Roll Rate Damping ==
  alpha : Inport
  del_lef : Inport  Port=2
  p : Inport  Port=3
  Add : Sum
  Constant : Constant
  Constant1 : Constant  Value=25
  Cy_p : Lookup_n-D  NumberOfTableDimensions=1  BreakpointsForDimension1=[-20, -15, -10, -5, 0, 5, 10, 15, 20, 25, 30, 35, 40, 45, 50, 55, 60, 70, 80, 90];  Table=aero_data.Cy_p  InternalRulePriority=Speed  RndMeth=Simplest
  Divide : Product  Inputs=*/
  Product : Product
  Product1 : Product
  Subtract : Sum  Inputs=+-
  del_Cy_p_lef : Lookup_n-D  NumberOfTableDimensions=1  BreakpointsForDimension1=[-20, -15, -10, -5, 0, 5, 10, 15, 20, 25, 30, 35, 40, 45];  Table=aero_data.del_Cy_p_lef  InternalRulePriority=Speed  RndMeth=Simplest
  Out1 : Outport
  wires:
  alpha/1 -> del_Cy_p_lef/1, Cy_p/1
  del_Cy_p_lef/1 -> Product/1  "del_Cy_p_lef"
  Cy_p/1 -> Add/1
  del_lef/1 -> Divide/1
  Constant1/1 -> Divide/2
  Constant/1 -> Subtract/1
  Divide/1 -> Subtract/2
  Subtract/1 -> Product/2  "1 - del_lef/25"
  Product/1 -> Add/2
  Add/1 -> Product1/1
  p/1 -> Product1/2
  Product1/1 -> Out1/1

== system F16_Model_/AeroForcesMoments/Aerodynamics/C_y/Rudder Adjustment ==
  "Cy(alpha, beta)" : Inport
  alpha : Inport  Port=2
  beta : Inport  Port=3
  del_r : Inport  Port=4
  Cy_del_r_30 : Lookup_n-D  BreakpointsForDimension1=[-20, -15, -10, -5, 0, 5, 10, 15, 20, 25, 30, 35, 40, 45, 50, 55, 60, 70, 80, 90];  BreakpointsForDimension2=[-30, -25, -20, -15, -10, -8, -6, -4, -2, 0, 2, 4, 6, 8, 10, 15, 20, 25, 30];  Table=aero_data.Cy_r_del_r_30  InternalRulePriority=Speed  RndMeth=Simplest
      settings: InputPortMap=u0,u1
  Product1 : Product
  Subtract : Sum  Inputs=+-
  Out1 : Outport
  wires:
  "Cy(alpha, beta)"/1 -> Subtract/2
  del_r/1 -> Product1/1
  Subtract/1 -> Product1/2
  Cy_del_r_30/1 -> Subtract/1  "Cy_del_r_30"
  alpha/1 -> Cy_del_r_30/1
  beta/1 -> Cy_del_r_30/2
  Product1/1 -> Out1/1

== system F16_Model_/AeroForcesMoments/Aerodynamics/C_y/Yaw Rate Damping ==
  alpha : Inport
  del_lef : Inport  Port=2
  r : Inport  Port=3
  Add : Sum
  Constant : Constant
  Constant1 : Constant  Value=25
  Cy_r : Lookup_n-D  NumberOfTableDimensions=1  BreakpointsForDimension1=[-20, -15, -10, -5, 0, 5, 10, 15, 20, 25, 30, 35, 40, 45, 50, 55, 60, 70, 80, 90];  Table=aero_data.Cy_r  InternalRulePriority=Speed  RndMeth=Simplest
  Divide : Product  Inputs=*/
  Product : Product
  Product1 : Product
  Subtract : Sum  Inputs=+-
  del_Cy_r_lef : Lookup_n-D  NumberOfTableDimensions=1  BreakpointsForDimension1=[-20, -15, -10, -5, 0, 5, 10, 15, 20, 25, 30, 35, 40, 45];  Table=aero_data.del_Cy_r_lef  InternalRulePriority=Speed  RndMeth=Simplest
  Out1 : Outport
  wires:
  Cy_r/1 -> Add/1
  alpha/1 -> del_Cy_r_lef/1, Cy_r/1
  del_Cy_r_lef/1 -> Product/1
  del_lef/1 -> Divide/1
  Divide/1 -> Subtract/2
  Subtract/1 -> Product/2  "1 - del_lef/25"
  Constant/1 -> Subtract/1
  Constant1/1 -> Divide/2
  Product/1 -> Add/2
  Add/1 -> Product1/1
  r/1 -> Product1/2
  Product1/1 -> Out1/1

== system F16_Model_/AeroForcesMoments/Aerodynamics/Cl/Aileron Adjustment ==
  alpha : Inport
  beta : Inport  Port=2
  del_lef : Inport  Port=3
  del_a : Inport  Port=4
  Add : Sum
  Cl_del_a_20 : Lookup_n-D  BreakpointsForDimension1=[-20, -15, -10, -5, 0, 5, 10, 15, 20, 25, 30, 35, 40, 45, 50, 55, 60, 70, 80, 90];  BreakpointsForDimension2=[-30, -25, -20, -15, -10, -8, -6, -4, -2, 0, 2, 4, 6, 8, 10, 15, 20, 25, 30];  Table=aero_data.Cl_del_a_20  InternalRulePriority=Speed  RndMeth=Simplest
      settings: InputPortMap=u0,u1
  Cl_del_a_20_lef : Lookup_n-D  BreakpointsForDimension1=[-20, -15, -10, -5, 0, 5, 10, 15, 20, 25, 30, 35, 40, 45];  BreakpointsForDimension2=[-30, -25, -20, -15, -10, -8, -6, -4, -2, 0, 2, 4, 6, 8, 10, 15, 20, 25, 30];  Table=aero_data.Cl_del_a_20_lef  InternalRulePriority=Speed  RndMeth=Simplest
      settings: InputPortMap=u0,u1
  Cl_del_h_0 : Lookup_n-D  BreakpointsForDimension1=[-20, -15, -10, -5, 0, 5, 10, 15, 20, 25, 30, 35, 40, 45, 50, 55, 60, 70, 80, 90];  BreakpointsForDimension2=[-30, -25, -20, -15, -10, -8, -6, -4, -2, 0, 2, 4, 6, 8, 10, 15, 20, 25, 30];  Table=aero_data.Cl_del_h_0  InternalRulePriority=Speed  RndMeth=Simplest
      settings: InputPortMap=u0,u1
  Cl_lef1 : Lookup_n-D  BreakpointsForDimension1=[-20, -15, -10, -5, 0, 5, 10, 15, 20, 25, 30, 35, 40, 45];  BreakpointsForDimension2=[-30, -25, -20, -15, -10, -8, -6, -4, -2, 0, 2, 4, 6, 8, 10, 15, 20, 25, 30];  Table=aero_data.Cl_lef  InternalRulePriority=Speed  RndMeth=Simplest
      settings: InputPortMap=u0,u1
  Constant : Constant
  Multiply : Gain  Gain=0.04
  Multiply1 : Gain  Gain=0.05
  Product : Product
  Product1 : Product
  Subtract : Sum  Inputs=+--
  Subtract1 : Sum  Inputs=+-
  Subtract2 : Sum  Inputs=+-
  Out1 : Outport
  wires:
  alpha/1 -> Cl_del_a_20_lef/1, Cl_lef1/1, Cl_del_h_0/1, Cl_del_a_20/1
  Cl_del_a_20/1 -> Subtract1/1
  beta/1 -> Cl_del_a_20/2, Cl_del_h_0/2, Cl_del_a_20_lef/2, Cl_lef1/2
  Cl_del_h_0/1 -> Subtract1/2
  Subtract1/1 -> Add/1, Subtract/3
  Cl_del_a_20_lef/1 -> Subtract/1
  Cl_lef1/1 -> Subtract/2
  Subtract/1 -> Product/1
  Constant/1 -> Subtract2/1
  Multiply/1 -> Subtract2/2
  del_lef/1 -> Multiply/1
  Subtract2/1 -> Product/2
  Product/1 -> Add/2
  Add/1 -> Product1/1
  del_a/1 -> Multiply1/1
  Multiply1/1 -> Product1/2
  Product1/1 -> Out1/1

== system F16_Model_/AeroForcesMoments/Aerodynamics/Cl/Leading Edge Flap Adjustment ==
  alpha : Inport
  beta : Inport  Port=2
  del_lef : Inport  Port=3
  Cl_del_h_0 : Lookup_n-D  BreakpointsForDimension1=[-20, -15, -10, -5, 0, 5, 10, 15, 20, 25, 30, 35, 40, 45, 50, 55, 60, 70, 80, 90];  BreakpointsForDimension2=[-30, -25, -20, -15, -10, -8, -6, -4, -2, 0, 2, 4, 6, 8, 10, 15, 20, 25, 30];  Table=aero_data.Cl_del_h_0  InternalRulePriority=Speed  RndMeth=Simplest
      settings: InputPortMap=u0,u1
  Cl_lef : Lookup_n-D  BreakpointsForDimension1=[-20, -15, -10, -5, 0, 5, 10, 15, 20, 25, 30, 35, 40, 45];  BreakpointsForDimension2=[-30, -25, -20, -15, -10, -8, -6, -4, -2, 0, 2, 4, 6, 8, 10, 15, 20, 25, 30];  Table=aero_data.Cl_lef  InternalRulePriority=Speed  RndMeth=Simplest
      settings: InputPortMap=u0,u1
  Constant : Constant
  Multiply : Gain  Gain=0.04
  Product : Product
  Subtract : Sum  Inputs=+-
  Subtract1 : Sum  Inputs=+-
  Out1 : Outport
  wires:
  alpha/1 -> Cl_del_h_0/1, Cl_lef/1
  Cl_lef/1 -> Subtract1/1
  Cl_del_h_0/1 -> Subtract1/2
  beta/1 -> Cl_del_h_0/2, Cl_lef/2
  del_lef/1 -> Multiply/1
  Constant/1 -> Subtract/1
  Multiply/1 -> Subtract/2
  Subtract/1 -> Product/2
  Subtract1/1 -> Product/1
  Product/1 -> Out1/1

== system F16_Model_/AeroForcesMoments/Aerodynamics/Cl/Roll Rate Damping ==
  alpha : Inport
  del_lef : Inport  Port=2
  p : Inport  Port=3
  Add : Sum
  Constant : Constant
  Constant1 : Constant  Value=25
  Cz_p : Lookup_n-D  NumberOfTableDimensions=1  BreakpointsForDimension1=[-20, -15, -10, -5, 0, 5, 10, 15, 20, 25, 30, 35, 40, 45, 50, 55, 60, 70, 80, 90];  Table=aero_data.Cl_p  InternalRulePriority=Speed  RndMeth=Simplest
  Divide : Product  Inputs=*/
  Product : Product
  Product1 : Product
  Subtract : Sum  Inputs=+-
  del_Cz_p_lef : Lookup_n-D  NumberOfTableDimensions=1  BreakpointsForDimension1=[-20, -15, -10, -5, 0, 5, 10, 15, 20, 25, 30, 35, 40, 45];  Table=aero_data.del_Cl_p_lef  InternalRulePriority=Speed  RndMeth=Simplest
  Out1 : Outport
  wires:
  alpha/1 -> del_Cz_p_lef/1, Cz_p/1
  del_Cz_p_lef/1 -> Product/1  "del_Cz_p_lef"
  Cz_p/1 -> Add/1
  del_lef/1 -> Divide/1
  Constant1/1 -> Divide/2
  Constant/1 -> Subtract/1
  Divide/1 -> Subtract/2
  Subtract/1 -> Product/2  "1 - del_lef/25"
  Product/1 -> Add/2
  Add/1 -> Product1/1
  p/1 -> Product1/2
  Product1/1 -> Out1/1

== system F16_Model_/AeroForcesMoments/Aerodynamics/Cl/Rudder Adjustment ==
  alpha : Inport
  beta : Inport  Port=2
  del_r : Inport  Port=3
  Cl_del_a_20 : Lookup_n-D  BreakpointsForDimension1=[-20, -15, -10, -5, 0, 5, 10, 15, 20, 25, 30, 35, 40, 45, 50, 55, 60, 70, 80, 90];  BreakpointsForDimension2=[-30, -25, -20, -15, -10, -8, -6, -4, -2, 0, 2, 4, 6, 8, 10, 15, 20, 25, 30];  Table=aero_data.Cl_del_r_30  InternalRulePriority=Speed  RndMeth=Simplest
      settings: InputPortMap=u0,u1
  Cl_del_h_0 : Lookup_n-D  BreakpointsForDimension1=[-20, -15, -10, -5, 0, 5, 10, 15, 20, 25, 30, 35, 40, 45, 50, 55, 60, 70, 80, 90];  BreakpointsForDimension2=[-30, -25, -20, -15, -10, -8, -6, -4, -2, 0, 2, 4, 6, 8, 10, 15, 20, 25, 30];  Table=aero_data.Cl_del_h_0  InternalRulePriority=Speed  RndMeth=Simplest
      settings: InputPortMap=u0,u1
  Multiply : Gain  Gain=1/30
  Product : Product
  Subtract : Sum  Inputs=+-
  Out1 : Outport
  wires:
  beta/1 -> Cl_del_h_0/2, Cl_del_a_20/2
  Cl_del_h_0/1 -> Subtract/2
  Cl_del_a_20/1 -> Subtract/1
  alpha/1 -> Cl_del_h_0/1, Cl_del_a_20/1
  del_r/1 -> Multiply/1
  Subtract/1 -> Product/1
  Multiply/1 -> Product/2
  Product/1 -> Out1/1

== system F16_Model_/AeroForcesMoments/Aerodynamics/Cl/Yaw Rate Damping ==
  alpha : Inport
  del_lef : Inport  Port=2
  r : Inport  Port=3
  Add : Sum
  Cl_r : Lookup_n-D  NumberOfTableDimensions=1  BreakpointsForDimension1=[-20, -15, -10, -5, 0, 5, 10, 15, 20, 25, 30, 35, 40, 45, 50, 55, 60, 70, 80, 90];  Table=aero_data.Cl_r  InternalRulePriority=Speed  RndMeth=Simplest
  Constant : Constant
  Constant1 : Constant  Value=25
  Divide : Product  Inputs=*/
  Product : Product
  Product1 : Product
  Subtract : Sum  Inputs=+-
  del_Cl_r_lef : Lookup_n-D  NumberOfTableDimensions=1  BreakpointsForDimension1=[-20, -15, -10, -5, 0, 5, 10, 15, 20, 25, 30, 35, 40, 45];  Table=aero_data.del_Cl_r_lef  InternalRulePriority=Speed  RndMeth=Simplest
  Out1 : Outport
  wires:
  Cl_r/1 -> Add/1
  alpha/1 -> del_Cl_r_lef/1, Cl_r/1
  del_Cl_r_lef/1 -> Product/1
  del_lef/1 -> Divide/1
  Divide/1 -> Subtract/2
  Subtract/1 -> Product/2  "1 - del_lef/25"
  Constant/1 -> Subtract/1
  Constant1/1 -> Divide/2
  Product/1 -> Add/2
  Add/1 -> Product1/1
  r/1 -> Product1/2
  Product1/1 -> Out1/1

== system F16_Model_/AeroForcesMoments/Aerodynamics/Cm/Leading Edge Flap Adjustment ==
  alpha : Inport
  beta : Inport  Port=2
  del_lef : Inport  Port=3
  Cm_del_h_0 : Lookup_n-D  BreakpointsForDimension1=[-20, -15, -10, -5, 0, 5, 10, 15, 20, 25, 30, 35, 40, 45, 50, 55, 60, 70, 80, 90];  BreakpointsForDimension2=[-30, -25, -20, -15, -10, -8, -6, -4, -2, 0, 2, 4, 6, 8, 10, 15, 20, 25, 30];  Table=aero_data.Cm_del_h_0  InternalRulePriority=Speed  RndMeth=Simplest
      settings: InputPortMap=u0,u1
  Cm_lef : Lookup_n-D  BreakpointsForDimension1=[-20, -15, -10, -5, 0, 5, 10, 15, 20, 25, 30, 35, 40, 45];  BreakpointsForDimension2=[-30, -25, -20, -15, -10, -8, -6, -4, -2, 0, 2, 4, 6, 8, 10, 15, 20, 25, 30];  Table=aero_data.Cm_lef  InternalRulePriority=Speed  RndMeth=Simplest
      settings: InputPortMap=u0,u1
  Constant : Constant
  Constant1 : Constant  Value=25
  Divide : Product  Inputs=*/
  Product : Product
  Subtract : Sum  Inputs=+-
  Subtract1 : Sum  Inputs=+-
  Out1 : Outport
  wires:
  alpha/1 -> Cm_lef/1, Cm_del_h_0/1
  Subtract/1 -> Product/1
  Cm_del_h_0/1 -> Subtract/2  "Cm_del_h_0"
  Product/1 -> Out1/1
  Cm_lef/1 -> Subtract/1  "Cm_lef"
  beta/1 -> Cm_lef/2, Cm_del_h_0/2
  del_lef/1 -> Divide/1
  Constant1/1 -> Divide/2
  Constant/1 -> Subtract1/1
  Divide/1 -> Subtract1/2
  Subtract1/1 -> Product/2

== system F16_Model_/AeroForcesMoments/Aerodynamics/Cm/Pitching Rate Damping ==
  note: (c_bar*q)/(2*V)
  alpha : Inport
  q : Inport  Port=2
  V : Inport  Port=3
  del_lef : Inport  Port=4
  Add : Sum
  Cmq : Lookup_n-D  NumberOfTableDimensions=1  BreakpointsForDimension1=[-20, -15, -10, -5, 0, 5, 10, 15, 20, 25, 30, 35, 40, 45, 50, 55, 60, 70, 80, 90];  Table=aero_data.Cmq  InternalRulePriority=Speed  RndMeth=Simplest
  Constant1 : Constant  Value=2
  Constant2 : Constant
  Constant3 : Constant  Value=25
  Divide : Product  Inputs=*/
  Divide1 : Product  Inputs=*/
  Product{,1..3} (4 alike) : Product
  Subtract1 : Sum  Inputs=+-
  cbar : Constant  Value=c_bar
  delCmq_lef : Lookup_n-D  NumberOfTableDimensions=1  BreakpointsForDimension1=[-20, -15, -10, -5, 0, 5, 10, 15, 20, 25, 30, 35, 40, 45];  Table=aero_data.del_Cmq_lef  InternalRulePriority=Speed  RndMeth=Simplest
  Out1 : Outport
  wires:
  Add/1 -> Product2/1
  Product3/1 -> Add/2
  Cmq/1 -> Add/1  "Cmq"
  delCmq_lef/1 -> Product3/1  "delCmq_lef"
  Product2/1 -> Out1/1
  alpha/1 -> Cmq/1, delCmq_lef/1
  q/1 -> Product/1
  cbar/1 -> Product/2
  Product/1 -> Divide/1
  Constant1/1 -> Product1/1
  V/1 -> Product1/2
  Product1/1 -> Divide/2
  Divide/1 -> Product2/2
  Constant2/1 -> Subtract1/1
  Divide1/1 -> Subtract1/2
  Subtract1/1 -> Product3/2
  del_lef/1 -> Divide1/1
  Constant3/1 -> Divide1/2

== system F16_Model_/AeroForcesMoments/Aerodynamics/Cm/Speed Brake ==
  alpha : Inport
  del_sb : Inport  Port=2
  Constant : Constant  Value=60
  Divide : Product  Inputs=*/
  Product : Product
  delCm_sb : Lookup_n-D  NumberOfTableDimensions=1  BreakpointsForDimension1=[-20, -15, -10, -5, 0, 5, 10, 15, 20, 25, 30, 35, 40, 45, 50, 55, 60, 70, 80, 90];  Table=aero_data.del_Cm_sb  InternalRulePriority=Speed  RndMeth=Simplest
  Out1 : Outport
  wires:
  delCm_sb/1 -> Product/1  "delCm_sb"
  Product/1 -> Out1/1
  alpha/1 -> delCm_sb/1
  del_sb/1 -> Divide/1
  Constant/1 -> Divide/2
  Divide/1 -> Product/2

== system F16_Model_/AeroForcesMoments/Aerodynamics/Cn/Aileron Adjustment ==
  alpha : Inport
  beta : Inport  Port=2
  del_lef : Inport  Port=3
  del_a : Inport  Port=4
  Add : Sum
  Cn_del_a_20 : Lookup_n-D  BreakpointsForDimension1=[-20, -15, -10, -5, 0, 5, 10, 15, 20, 25, 30, 35, 40, 45, 50, 55, 60, 70, 80, 90];  BreakpointsForDimension2=[-30, -25, -20, -15, -10, -8, -6, -4, -2, 0, 2, 4, 6, 8, 10, 15, 20, 25, 30];  Table=aero_data.Cn_del_a_20  InternalRulePriority=Speed  RndMeth=Simplest
      settings: InputPortMap=u0,u1
  Cn_del_a_20_lef : Lookup_n-D  BreakpointsForDimension1=[-20, -15, -10, -5, 0, 5, 10, 15, 20, 25, 30, 35, 40, 45];  BreakpointsForDimension2=[-30, -25, -20, -15, -10, -8, -6, -4, -2, 0, 2, 4, 6, 8, 10, 15, 20, 25, 30];  Table=aero_data.Cn_del_a_20_lef  InternalRulePriority=Speed  RndMeth=Simplest
      settings: InputPortMap=u0,u1
  Cn_del_h_0 : Lookup_n-D  BreakpointsForDimension1=[-20, -15, -10, -5, 0, 5, 10, 15, 20, 25, 30, 35, 40, 45, 50, 55, 60, 70, 80, 90];  BreakpointsForDimension2=[-30, -25, -20, -15, -10, -8, -6, -4, -2, 0, 2, 4, 6, 8, 10, 15, 20, 25, 30];  Table=aero_data.Cn_del_h_0  InternalRulePriority=Speed  RndMeth=Simplest
      settings: InputPortMap=u0,u1
  Cn_lef : Lookup_n-D  BreakpointsForDimension1=[-20, -15, -10, -5, 0, 5, 10, 15, 20, 25, 30, 35, 40, 45];  BreakpointsForDimension2=[-30, -25, -20, -15, -10, -8, -6, -4, -2, 0, 2, 4, 6, 8, 10, 15, 20, 25, 30];  Table=aero_data.Cn_lef  InternalRulePriority=Speed  RndMeth=Simplest
      settings: InputPortMap=u0,u1
  Constant : Constant
  Multiply : Gain  Gain=0.04
  Multiply1 : Gain  Gain=0.05
  Product : Product
  Product1 : Product
  Subtract : Sum  Inputs=+--
  Subtract1 : Sum  Inputs=+-
  Subtract2 : Sum  Inputs=+-
  Out1 : Outport
  wires:
  alpha/1 -> Cn_del_a_20_lef/1, Cn_lef/1, Cn_del_h_0/1, Cn_del_a_20/1
  Cn_del_a_20/1 -> Subtract1/1
  beta/1 -> Cn_del_a_20/2, Cn_del_h_0/2, Cn_del_a_20_lef/2, Cn_lef/2
  Cn_del_h_0/1 -> Subtract1/2
  Subtract1/1 -> Add/1, Subtract/3
  Cn_del_a_20_lef/1 -> Subtract/1
  Cn_lef/1 -> Subtract/2
  Subtract/1 -> Product/1
  Constant/1 -> Subtract2/1
  Multiply/1 -> Subtract2/2
  del_lef/1 -> Multiply/1
  Subtract2/1 -> Product/2
  Product/1 -> Add/2
  Add/1 -> Product1/1
  del_a/1 -> Multiply1/1
  Multiply1/1 -> Product1/2
  Product1/1 -> Out1/1
